simulink model "basab_thalamocorticothalamicCkt"  (Simulink 7.3)
settings: Solver=ode4  StartTime=0.0  StopTime=60  FixedStep=.004  RelTol=1e-3
Description:
  | THE MODEL IS DESIGNED BY BASABDATTA SEN BHATTACHARYA
  | AND IS AN INTELLECTUAL PROPERTY OF THE UNIVERSITY OF ULSTER,
  | NORTHERN IRELAND, UK.
  | PLEASE CITE THE FOLLOWING PAPER WHEN USING THE MODEL IN YOUR WORK:
  | Sen Bhattacharya, Basabdatta, Coyle, Damien, Maguire, Liam:
  | "A thalamo-cortico-thalamic neural mass model to study alpha rhythms in Alzheimer's
  | disease", Neural Networks (2011), doi:10.1016/j.neunet.2011.02.009.
settings Model: Creator=basabb  LastModifiedBy=basabb
settings DataIOCC: LimitDataPoints=off  SaveOutput=off  SignalLogging=off  SaveTime=off
settings DebuggingCC: SaveWithParameterizedLinksMsg=none  InheritedTsInSrcMsg=none  ModelReferenceDataLoggingMessage=none
settings RTWCC: IncludeERTFirstTime=on

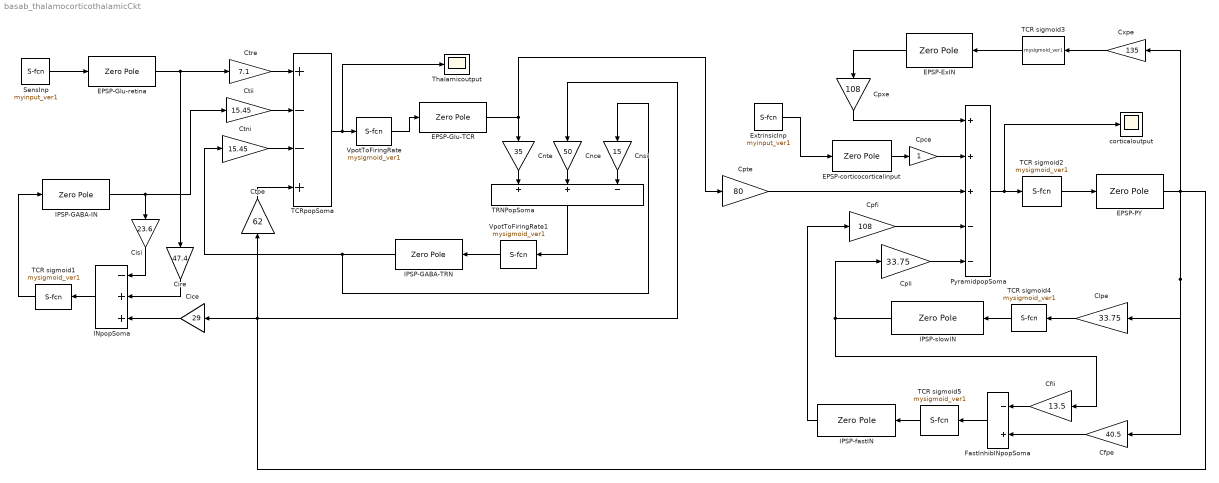
== system basab_thalamocorticothalamicCkt ==
  Cfli : Gain  Gain=13.5  ParameterDataType=fixdt(1, 16)  ParameterScaling=2^0  OutDataType=fixdt(1, 16)  OutScaling=2^0
  Cfpe : Gain  Gain=40.5  ParameterDataType=fixdt(1, 16)  ParameterScaling=2^0  OutDataType=fixdt(1, 16)  OutScaling=2^0
  Cice : Gain  Gain=29  ParameterDataType=fixdt(1, 16)  ParameterScaling=2^0  OutDataType=fixdt(1, 16)  OutScaling=2^0
  Cire : Gain  Gain=47.4  ParameterDataType=fixdt(1, 16)  ParameterScaling=2^0  OutDataType=fixdt(1, 16)  OutScaling=2^0
  Cisi : Gain  Gain=23.6  ParameterDataType=fixdt(1, 16)  ParameterScaling=2^0  OutDataType=fixdt(1, 16)  OutScaling=2^0
  Clpe : Gain  Gain=33.75  ParameterDataType=fixdt(1, 16)  ParameterScaling=2^0  OutDataType=fixdt(1, 16)  OutScaling=2^0
  Cnce : Gain  Gain=50  ParameterDataType=fixdt(1, 16)  ParameterScaling=2^0  OutDataType=fixdt(1, 16)  OutScaling=2^0
  Cnsi : Gain  Gain=15  ParameterDataType=fixdt(1, 16)  ParameterScaling=2^0  OutDataType=fixdt(1, 16)  OutScaling=2^0
  Cnte : Gain  Gain=35  ParameterDataType=fixdt(1, 16)  ParameterScaling=2^0  OutDataType=fixdt(1, 16)  OutScaling=2^0
  Cpce : Gain  ParameterDataType=fixdt(1, 16)  ParameterScaling=2^0  OutDataType=fixdt(1, 16)  OutScaling=2^0
  Cpfi : Gain  Gain=108  ParameterDataType=fixdt(1, 16)  ParameterScaling=2^0  OutDataType=fixdt(1, 16)  OutScaling=2^0
  Cpli : Gain  Gain=33.75  ParameterDataType=fixdt(1, 16)  ParameterScaling=2^0  OutDataType=fixdt(1, 16)  OutScaling=2^0
  Cpte : Gain  Gain=80  ParameterDataType=fixdt(1, 16)  ParameterScaling=2^0  OutDataType=fixdt(1, 16)  OutScaling=2^0
  Cpxe : Gain  Gain=108  ParameterDataType=fixdt(1, 16)  ParameterScaling=2^0  OutDataType=fixdt(1, 16)  OutScaling=2^0
  Ctii : Gain  Gain=15.45  ParameterDataType=fixdt(1, 16)  ParameterScaling=2^0  OutDataType=fixdt(1, 16)  OutScaling=2^0
  Ctni : Gain  Gain=15.45  ParameterDataType=fixdt(1, 16)  ParameterScaling=2^0  OutDataType=fixdt(1, 16)  OutScaling=2^0
  Ctpe : Gain  Gain=62  ParameterDataType=fixdt(1, 16)  ParameterScaling=2^0  OutDataType=fixdt(1, 16)  OutScaling=2^0
  Ctre : Gain  Gain=7.1  ParameterDataType=fixdt(1, 16)  ParameterScaling=2^0  OutDataType=fixdt(1, 16)  OutScaling=2^0
  Cxpe : Gain  Gain=135  ParameterDataType=fixdt(1, 16)  ParameterScaling=2^0  OutDataType=fixdt(1, 16)  OutScaling=2^0
  EPSP-ExIN : ZeroPole  Zeros=[]  Poles=[-40 -40]  Gain=[40* 0.0027]
  EPSP-Glu-TCR : ZeroPole  Zeros=[]  Poles=[-100 -100]  Gain=[0.00325*100]
  EPSP-Glu-retina : ZeroPole  Zeros=[]  Poles=[-100 -100]  Gain=[0.00325*100]
  EPSP-PY : ZeroPole  Zeros=[]  Poles=[-40 -40]  Gain=[40* 0.0027]
  EPSP-corticocorticalinput : ZeroPole  Zeros=[]  Poles=[-40 -40]  Gain=[40* 0.0027]
  ExtrinsicInp : M-S-Function  Description=|  FunctionName=myinput_ver1  Parameters=30,5,60000,1
      | Input to the model with or without noise. The order of input parameters in the Dialog box is:                      
      | mean, standard deviation, length of signal,flag,constant.                                                          
      | If flag is 0, the input is a constant devoid of any noise. However, if flag is 1, the noise is added to the signal.
      mask Display: plot(312+randn(1,25))
  FastInhibINpopSoma : Sum  Inputs=-+  CollapseMode=Specified dimension  CollapseDim=4  OutDataType=fixdt(1, 16)  OutScaling=2^-10
  INpopSoma : Sum  Inputs=-++  CollapseMode=Specified dimension  CollapseDim=4  OutDataType=fixdt(1, 16)  OutScaling=2^-10
  IPSP-GABA-IN : ZeroPole  Zeros=[]  Poles=[-40 -40]  Gain=[0.022*40]
  IPSP-GABA-TRN : ZeroPole  Zeros=[]  Poles=[-40 -40]  Gain=[0.022*40]
  IPSP-fastIN : ZeroPole  Zeros=[]  Poles=[-300 -300]  Gain=[300*0.039]
  IPSP-slowIN : ZeroPole  Zeros=[]  Poles=[-20 -20]  Gain=[20*0.0045]
  PyramidpopSoma : Sum  Inputs=+++--  CollapseMode=Specified dimension  CollapseDim=4  OutDataType=fixdt(1, 16)  OutScaling=2^-10
  SensInp : M-S-Function  Description=|  FunctionName=myinput_ver1  Parameters=11,5,60000,1
      | Input to the model with or without noise. The order of input parameters in the Dialog box is:                      
      | mean, standard deviation, length of signal,flag,constant.                                                          
      | If flag is 0, the input is a constant devoid of any noise. However, if flag is 1, the noise is added to the signal.
      mask Display: plot(312+randn(1,25))
  TCR sigmoid{1..5} (5 alike) : M-S-Function  FunctionName=mysigmoid_ver1  Parameters=2.5,560,0.006
      mask Display: plot(1./(1+exp(-0.75.*([1:25]-12))))
  TCRpopSoma : Sum  Inputs=+--+  CollapseMode=Specified dimension  CollapseDim=4  OutDataType=fixdt(1, 16)  OutScaling=2^-10
  TRNPopSoma : Sum  Inputs=++-  CollapseMode=Specified dimension  CollapseDim=4  OutDataType=fixdt(1, 16)  OutScaling=2^-10
  Thalamicoutput : Scope
      settings: TickLabels=on  TimeRange=60  YMin=0.00016  YMax=0.000171  SaveName=thalamicoutput  SampleInput=on  SampleTime=0.004
  VpotToFiringRate : M-S-Function  FunctionName=mysigmoid_ver1  Parameters=2.5,560,0.006
      mask Display: plot(1./(1+exp(-0.75.*([1:25]-12))))
  VpotToFiringRate1 : M-S-Function  FunctionName=mysigmoid_ver1  Parameters=2.5,560,0.006
      mask Display: plot(1./(1+exp(-0.75.*([1:25]-12))))
  corticaloutput : Scope
      settings: YMin=0.00865  YMax=0.008825  SaveName=corticaloutput  SampleInput=on  SampleTime=0.004
  wires:
  Ctre/1 -> TCRpopSoma/1
  SensInp/1 -> EPSP-Glu-retina/1
  EPSP-Glu-retina/1 -> Ctre/1, Cire/1
  TCRpopSoma/1 -> VpotToFiringRate/1, Thalamicoutput/1
  INpopSoma/1 -> TCR sigmoid1/1
  Cire/1 -> INpopSoma/2
  TCR sigmoid1/1 -> IPSP-GABA-IN/1
  IPSP-GABA-IN/1 -> Ctii/1, Cisi/1
  TRNPopSoma/1 -> VpotToFiringRate1/1
  VpotToFiringRate/1 -> EPSP-Glu-TCR/1
  Cnte/1 -> TRNPopSoma/1
  VpotToFiringRate1/1 -> IPSP-GABA-TRN/1
  IPSP-GABA-TRN/1 -> Ctni/1, Cnsi/1
  Cnce/1 -> TRNPopSoma/2
  Ctii/1 -> TCRpopSoma/2
  Ctni/1 -> TCRpopSoma/3
  Ctpe/1 -> TCRpopSoma/4
  Cisi/1 -> INpopSoma/1
  Cice/1 -> INpopSoma/3
  Cnsi/1 -> TRNPopSoma/3
  EPSP-Glu-TCR/1 -> Cnte/1, Cpte/1
  PyramidpopSoma/1 -> TCR sigmoid2/1, corticaloutput/1
  TCR sigmoid2/1 -> EPSP-PY/1
  Cxpe/1 -> TCR sigmoid3/1
  TCR sigmoid3/1 -> EPSP-ExIN/1
  Clpe/1 -> TCR sigmoid4/1
  TCR sigmoid4/1 -> IPSP-slowIN/1
  IPSP-slowIN/1 -> Cpli/1, Cfli/1
  Cfli/1 -> FastInhibINpopSoma/1
  TCR sigmoid5/1 -> IPSP-fastIN/1
  IPSP-fastIN/1 -> Cpfi/1
  EPSP-ExIN/1 -> Cpxe/1
  EPSP-PY/1 -> Clpe/1, Cfpe/1, Cxpe/1, Ctpe/1, Cice/1, Cnce/1
  FastInhibINpopSoma/1 -> TCR sigmoid5/1
  Cfpe/1 -> FastInhibINpopSoma/2
  ExtrinsicInp/1 -> EPSP-corticocorticalinput/1
  Cpxe/1 -> PyramidpopSoma/1
  EPSP-corticocorticalinput/1 -> Cpce/1
  Cpfi/1 -> PyramidpopSoma/4
  Cpli/1 -> PyramidpopSoma/5
  Cpte/1 -> PyramidpopSoma/3
  Cpce/1 -> PyramidpopSoma/2
